simulink model "Idle_Stop_Control"  (R2018a)
settings: configuration reference "Config_Ctrl_Module" (kept outside this file)
PreLoadFcn:
  | HEV_Ctrl_V1_PreLoad
libraries: simulink x1
settings Model: DataDictionary=HEV_Ctrl_V1_Local_data.sldd  Creator=IAEC nishito  LastModifiedBy=E00026

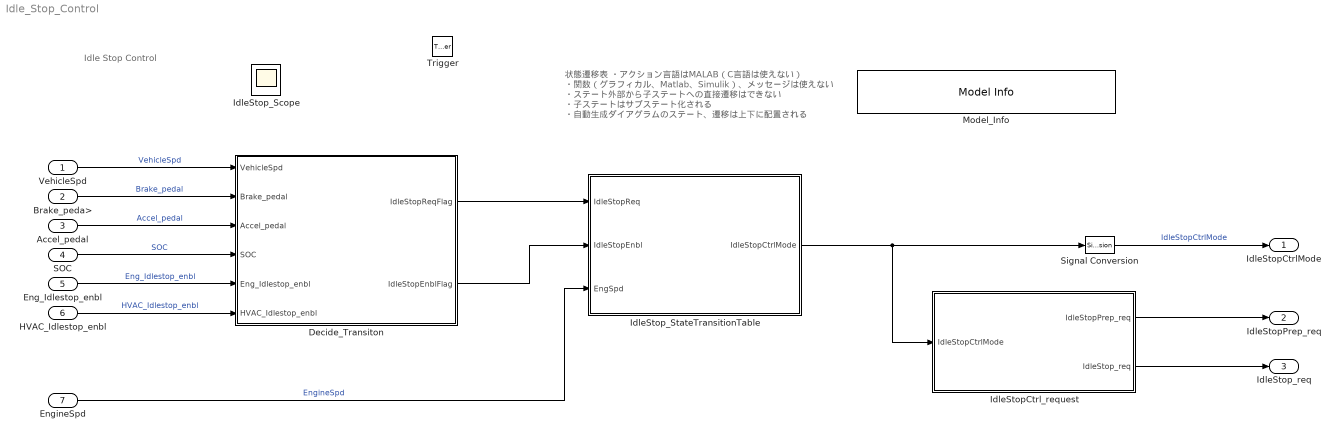
== system Idle_Stop_Control ==
  note: 状態遷移表
      | ・アクション言語はMALAB（C言語は使えない）
      | ・関数（グラフィカル、Matlab、Simulik）、メッセージは使えない
      | ・ステート外部から子ステートへの直接遷移はできない
      | ・子ステートはサブステート化される
      | ・自動生成ダイアグラムのステート、遷移は上下に配置される
  note: Idle Stop Control
  VehicleSpd : Inport  RequirementInfo={} %GIDa_72f7735f_1861_41c0_a3c3_402e3e844fc1  OutDataTypeStr=double  PortDimensions=1
  Brake_peda> : Inport  RequirementInfo={} %GIDa_eb069480_9703_4585_8fff_a42166b4aebb  Port=2  OutDataTypeStr=double  PortDimensions=1
  Accel_pedal : Inport  RequirementInfo={} %GIDa_c2aa2f20_ded1_4ed8_bb49_4c61baf6c527  Port=3  OutDataTypeStr=double  PortDimensions=1
  SOC : Inport  RequirementInfo={} %GIDa_2288a541_41c6_47f0_af5b_526a61592d01  Port=4  OutDataTypeStr=double  PortDimensions=1
  Eng_Idlestop_enbl : Inport  RequirementInfo={} %GIDa_52f2a631_deee_4b81_b109_144a38fb1d39  Port=5  OutDataTypeStr=boolean  PortDimensions=1
  HVAC_Idlestop_enbl : Inport  RequirementInfo={} %GIDa_a5979ef4_7306_49ba_b132_d6093500969e  Port=6  OutDataTypeStr=boolean  PortDimensions=1
  EngineSpd : Inport  RequirementInfo={} %GIDa_0144a9fc_2fd0_4446_b957_811392ba3fbb  Port=7  OutDataTypeStr=double  PortDimensions=1
  Trigger : TriggerPort  RequirementInfo={} %GIDa_12d1da28_9432_4f31_ab1a_c0ce181fbae1  TriggerType=function-call  VariantControl=Variant  PortDimensions=1  TriggerSignalSampleTime=[0.01,0]
  Decide_Transiton : Subsystem  RequirementInfo={} %GIDa_0f8c3e68_9d09_4b6b_9107_8d1ed7fa0379
  IdleStopCtrl_request : Subsystem  RequirementInfo={} %GIDa_43d550b6_444b_4df2_903c_66ed82cd3cc1
  IdleStop_StateTransitionTable : State Transition Table  RequirementInfo={} %GIDa_4a150023_0398_44b8_a842_f2e371cb155a  TreatAsAtomicUnit=on
  Model_Info : simulink/Model-Wide Utilities/Model Info  Frame=on  DisplayStringWithTags=|  HorizontalTextAlignment=Left  LeftAlignmentValue=0.02
      | Version  %<ModelVersion>
      | LastModifided by %<LastModifiedBy>  Date %<LastModificationDate>
      | Description  %<Description>
  Signal Conversion : SignalConversion  OverrideOpt=off
  IdleStopCtrlMode : Outport  RequirementInfo={} %GIDa_55c5f649_78ac_4ac9_b2e5_0d2ecf0ccf0d  OutDataTypeStr=double  PortDimensions=1
  IdleStopPrep_req : Outport  RequirementInfo={} %GIDa_26006239_a740_4660_838b_7c9264c716dc  Port=2  OutDataTypeStr=boolean  PortDimensions=1
  IdleStop_req : Outport  RequirementInfo={} %GIDa_f6c09664_3b1e_412f_baf0_3722afa6614f  Port=3  OutDataTypeStr=boolean  PortDimensions=1
  IdleStop_Scope : Scope
      settings: RequirementInfo={} %GIDa_1aa572e7_9fb2_4501_b2d6_c4ee76e73ea6
  wires:
  IdleStopCtrl_request/2(IdleStop_req) -> IdleStop_req/1
  IdleStop_StateTransitionTable/1(IdleStopCtrlMode) -> IdleStopCtrl_request/1(IdleStopCtrlMode), Signal Conversion/1
  Decide_Transiton/1(IdleStopReqFlag) -> IdleStop_StateTransitionTable/1(IdleStopReq)
  SOC/1 -> Decide_Transiton/4(SOC)  "SOC"
  HVAC_Idlestop_enbl/1 -> Decide_Transiton/6(HVAC_Idlestop_enbl)  "HVAC_Idlestop_enbl"
  IdleStopCtrl_request/1(IdleStopPrep_req) -> IdleStopPrep_req/1
  Decide_Transiton/2(IdleStopEnblFlag) -> IdleStop_StateTransitionTable/2(IdleStopEnbl)
  Eng_Idlestop_enbl/1 -> Decide_Transiton/5(Eng_Idlestop_enbl)  "Eng_Idlestop_enbl"
  Accel_pedal/1 -> Decide_Transiton/3(Accel_pedal)  "Accel_pedal"
  VehicleSpd/1 -> Decide_Transiton/1(VehicleSpd)  "VehicleSpd"
  Brake_peda>/1 -> Decide_Transiton/2(Brake_pedal)  "Brake_pedal"
  EngineSpd/1 -> IdleStop_StateTransitionTable/3(EngSpd)  "EngineSpd"
  Signal Conversion/1 -> IdleStopCtrlMode/1  "IdleStopCtrlMode"

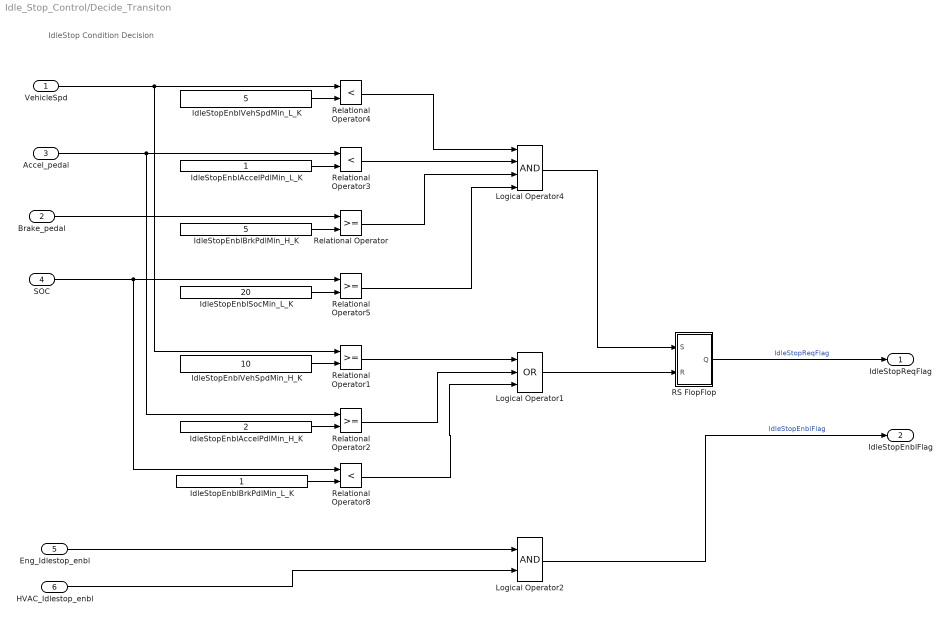
== system Idle_Stop_Control/Decide_Transiton ==
  note: IdleStop Condition Decision
  VehicleSpd : Inport  RequirementInfo={} %GIDa_2ab10adb_7032_4a2c_97a1_7bb0fb165e5e
  Brake_pedal : Inport  RequirementInfo={} %GIDa_47a88e33_5f43_40d8_bc0c_501364992970  Port=2
  Accel_pedal : Inport  RequirementInfo={} %GIDa_fef39789_89f0_45fa_8f85_6b84aa230c69  Port=3
  SOC : Inport  RequirementInfo={} %GIDa_55e6d60a_ee0f_44e0_a38d_ba6e2bf9dbe9  Port=4
  Eng_Idlestop_enbl : Inport  RequirementInfo={} %GIDa_91922d57_691f_49b7_a99e_006b578cf11a  Port=5
  HVAC_Idlestop_enbl : Inport  RequirementInfo={} %GIDa_566c9289_9246_4d35_932c_d372c551c6b7  Port=6
  IdleStopEnblAccelPdlMin_H_K : Constant  RequirementInfo={} %GIDa_806777b1_f885_41a3_adb0_404dc20a194f  Value=2
  IdleStopEnblAccelPdlMin_L_K : Constant  RequirementInfo={} %GIDa_c8f7521b_913c_432c_8051_26ac6e0716a2
  IdleStopEnblBrkPdlMin_H_K : Constant  RequirementInfo={} %GIDa_e5b7d4a4_8bf8_424f_97db_ebec4c30798e  Value=5
  IdleStopEnblBrkPdlMin_L_K : Constant  RequirementInfo={} %GIDa_272b3a83_c857_492d_b6b1_a02b8e962bbe
  IdleStopEnblSocMin_L_K : Constant  RequirementInfo={} %GIDa_3866ca77_8194_43de_88d7_1af354df2f6f  Value=20
  IdleStopEnblVehSpdMin_H_K : Constant  RequirementInfo={} %GIDa_161c09d4_4e2f_45d2_9a9e_7a4b2d014d7d  Value=10
  IdleStopEnblVehSpdMin_L_K : Constant  RequirementInfo={} %GIDa_e4333e70_a7b3_4f07_ad9b_22dc57ba8654  Value=5
  Logical Operator1 : Logic  RequirementInfo={} %GIDa_d1fd0692_7828_4595_92b3_37285b918121  Operator=OR  Inputs=3  AllPortsSameDT=off  OutDataTypeStr=boolean
  Logical Operator2 : Logic  RequirementInfo={} %GIDa_eeb31a4b_771d_490c_936b_5a131afa7c1f  AllPortsSameDT=off  OutDataTypeStr=boolean
  Logical Operator4 : Logic  RequirementInfo={} %GIDa_3a26ed1d_1d0a_42f0_8160_5b4b9b82dbe0  Inputs=4  AllPortsSameDT=off  OutDataTypeStr=boolean
  RS FlopFlop : Subsystem  RequirementInfo={} %GIDa_1f11bf5d_841d_4e55_8521_3cd2fe287deb
  Relational Operator : RelationalOperator  RequirementInfo={} %GIDa_fbc19323_8ea8_455f_abaf_2d6731ecb0a1  OutDataTypeStr=boolean  RndMeth=Nearest
  Relational Operator1 : RelationalOperator  RequirementInfo={} %GIDa_0f689cbf_b206_45df_8702_d5c355afebcd  OutDataTypeStr=boolean  RndMeth=Nearest
  Relational Operator2 : RelationalOperator  RequirementInfo={} %GIDa_badd182d_40d6_46ba_a742_a480e4b72dfc  OutDataTypeStr=boolean  RndMeth=Nearest
  Relational Operator3 : RelationalOperator  RequirementInfo={} %GIDa_9893dff2_f141_4666_ae75_117eb5370ef1  Operator=<  OutDataTypeStr=boolean  RndMeth=Nearest
  Relational Operator4 : RelationalOperator  RequirementInfo={} %GIDa_8927ae18_2ea7_4178_b421_484c846f4f3f  Operator=<  OutDataTypeStr=boolean  RndMeth=Nearest
  Relational Operator5 : RelationalOperator  RequirementInfo={} %GIDa_4427b0fb_90c4_45ec_83a1_a4700bbd409b  OutDataTypeStr=boolean  RndMeth=Nearest
  Relational Operator8 : RelationalOperator  RequirementInfo={} %GIDa_d6849958_8b19_4562_b9e4_7d2057c59388  Operator=<  OutDataTypeStr=boolean  RndMeth=Nearest
  IdleStopReqFlag : Outport  RequirementInfo={} %GIDa_9411fa9e_6f2a_4c7c_909d_f494b4c4f2c2
  IdleStopEnblFlag : Outport  RequirementInfo={} %GIDa_7a1f6d7a_c541_4108_a0bc_a841b5b25c82  Port=2
  wires:
  HVAC_Idlestop_enbl/1 -> Logical Operator2/2
  Eng_Idlestop_enbl/1 -> Logical Operator2/1
  Logical Operator2/1 -> IdleStopEnblFlag/1  "IdleStopEnblFlag"
  IdleStopEnblAccelPdlMin_L_K/1 -> Relational Operator3/2
  Relational Operator5/1 -> Logical Operator4/4
  SOC/1 -> Relational Operator5/1, Relational Operator8/1
  Relational Operator2/1 -> Logical Operator1/2
  IdleStopEnblAccelPdlMin_H_K/1 -> Relational Operator2/2
  Logical Operator4/1 -> RS FlopFlop/1(S)
  IdleStopEnblVehSpdMin_L_K/1 -> Relational Operator4/2
  VehicleSpd/1 -> Relational Operator4/1, Relational Operator1/1
  RS FlopFlop/1(Q) -> IdleStopReqFlag/1  "IdleStopReqFlag"
  IdleStopEnblSocMin_L_K/1 -> Relational Operator5/2
  Accel_pedal/1 -> Relational Operator2/1, Relational Operator3/1
  Relational Operator/1 -> Logical Operator4/3
  IdleStopEnblBrkPdlMin_H_K/1 -> Relational Operator/2
  Brake_pedal/1 -> Relational Operator/1
  Relational Operator4/1 -> Logical Operator4/1
  Relational Operator3/1 -> Logical Operator4/2
  Logical Operator1/1 -> RS FlopFlop/2(R)
  IdleStopEnblVehSpdMin_H_K/1 -> Relational Operator1/2
  IdleStopEnblBrkPdlMin_L_K/1 -> Relational Operator8/2
  Relational Operator1/1 -> Logical Operator1/1
  Relational Operator8/1 -> Logical Operator1/3

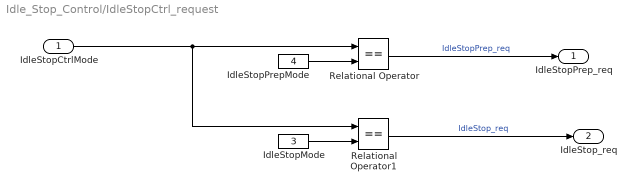
== system Idle_Stop_Control/IdleStopCtrl_request ==
  IdleStopCtrlMode : Inport  RequirementInfo={} %GIDa_1f284967_020f_4205_9752_6dfdc9c13a06
  IdleStopMode : Constant  RequirementInfo={} %GIDa_5e0ca651_d1c8_4f9d_9420_69ebc9aafafb  Value=3
  IdleStopPrepMode : Constant  RequirementInfo={} %GIDa_413a497d_dce0_4397_8719_5d8fd05e37eb  Value=4
  Relational Operator : RelationalOperator  RequirementInfo={} %GIDa_9d9c37b5_ea2b_406f_8f3d_fb66169759d4  Operator===  OutDataTypeStr=boolean  RndMeth=Simplest
  Relational Operator1 : RelationalOperator  RequirementInfo={} %GIDa_1724a5ed_5dcb_4ffd_b16b_83fc4d24ff06  Operator===  OutDataTypeStr=boolean  RndMeth=Simplest
  IdleStopPrep_req : Outport  RequirementInfo={} %GIDa_c88fe8dc_128e_4808_9ef1_67c706cdd285
  IdleStop_req : Outport  RequirementInfo={} %GIDa_88ed3775_e262_4a57_a1cf_ae30085eac21  Port=2
  wires:
  IdleStopPrepMode/1 -> Relational Operator/2
  Relational Operator/1 -> IdleStopPrep_req/1  "IdleStopPrep_req"
  IdleStopMode/1 -> Relational Operator1/2
  IdleStopCtrlMode/1 -> Relational Operator/1, Relational Operator1/1
  Relational Operator1/1 -> IdleStop_req/1  "IdleStop_req"

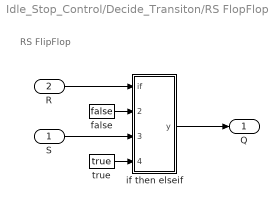
== system Idle_Stop_Control/Decide_Transiton/RS FlopFlop ==
  note: RS FlipFlop
  S : Inport  RequirementInfo={} %GIDa_0a6200b1_c4a0_4772_b261_301d0d627c45
  R : Inport  RequirementInfo={} %GIDa_6e1f103a_7746_4c5c_8128_9c2665cc449d  Port=2
  false : Constant  RequirementInfo={} %GIDa_b8d1b9da_7624_4755_882e_ea884b51896b  Value=false
  if then elseif : Subsystem  RequirementInfo={} %GIDa_b2bf0fbb_ebdd_4d78_ae41_ec1a71f47043  mask(if then elseif){}
  true : Constant  RequirementInfo={} %GIDa_feb0358c_0403_4a1b_8a43_a4add1c7c9f4  Value=true
  Q : Outport  RequirementInfo={} %GIDa_30c2e6ea_c9e6_431a_83b1_8a2226066ab0
  wires:
  S/1 -> if then elseif/3(elseif)
  R/1 -> if then elseif/1(if)
  if then elseif/1(y) -> Q/1
  false/1 -> if then elseif/2(then1)
  true/1 -> if then elseif/4(then2)

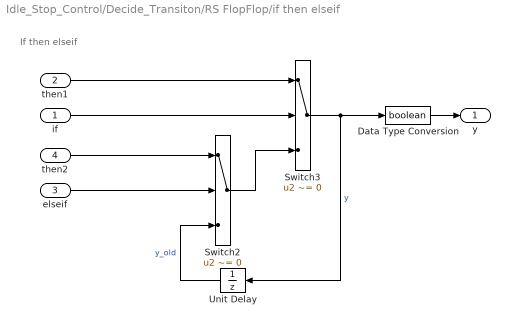
== system Idle_Stop_Control/Decide_Transiton/RS FlopFlop/if then elseif ==
  note: If then elseif
  if : Inport  RequirementInfo={} %GIDa_a06445fc_5d96_4bb4_b90a_65ade8082873
  then1 : Inport  RequirementInfo={} %GIDa_793bcde2_ca84_4662_961f_9b99bee5138c  Port=2
  elseif : Inport  RequirementInfo={} %GIDa_3058ce07_9bdf_4832_8ef2_ce84ef01be25  Port=3
  then2 : Inport  RequirementInfo={} %GIDa_fd0e4a57_410b_4495_b647_ecf5be5ab035  Port=4
  Data Type Conversion : DataTypeConversion  RequirementInfo={} %GIDa_04e57f06_0282_4d92_a01d_4e1bec4290de  OutDataTypeStr=boolean
  Switch2 : Switch  RequirementInfo={} %GIDa_1351dd5c_486a_460b_ba05_1fbf138bbcb6  Criteria=u2 ~= 0  Threshold=0.5  SaturateOnIntegerOverflow=on
      settings: AttributesFormatString=<%<Criteria>>
  Switch3 : Switch  RequirementInfo={} %GIDa_4fa8a9f2_3ad9_4cc8_bb0d_ea07fea45472  Criteria=u2 ~= 0  Threshold=0.5  SaturateOnIntegerOverflow=on
      settings: AttributesFormatString=<%<Criteria>>
  Unit Delay : UnitDelay  RequirementInfo={} %GIDa_94b45ce3_2546_4a04_8f73_a58228ae89e6  SampleTime=-1
      settings: AttributesFormatString=<initial=%<X0>>\n<tsample=%<SampleTime>>
  y : Outport  RequirementInfo={} %GIDa_4d4551a4_f4ea_480d_b486_6b8dd17e1939
  wires:
  Data Type Conversion/1 -> y/1
  Switch2/1 -> Switch3/3
  if/1 -> Switch3/2
  Unit Delay/1 -> Switch2/3  "y_old"
  Switch3/1 -> Data Type Conversion/1, Unit Delay/1  "y"
  then1/1 -> Switch3/1
  elseif/1 -> Switch2/2
  then2/1 -> Switch2/1

== stateflow chart Idle_Stop_Control/IdleStop_StateTransitionTable ==
  state EngineStop
    en:
    IdleStopCtrlMode=0;
  state IdleStop
    en:
    IdleStopCtrlMode=1;
  state EngineStart_Tran
    en:
    IdleStopCtrlMode=2;
  state IdleStopWait_Tran
    en:
    IdleStopCtrlMode=3;
  state IdleStopPrepare
    en:
    IdleStopCtrlMode=4;
  state EngineRun
    en:
    IdleStopCtrlMode=5;
  (default) -> EngineStop
  (junction 32) -> EngineStop
  (junction 52) -> (junction 32)
  EngineStop -> (junction 70) : [EngSpd>300]% Engine run cond
  (junction 70) -> (junction 28)
  (junction 65) -> IdleStop
  (junction 67) -> (junction 65)
  IdleStop -> EngineStart_Tran : [~IdleStopReq]% IdleStop end cond.
  EngineStart_Tran -> IdleStop [order 2] : [IdleStopReq]% IdleStop restart cond.
  EngineStart_Tran -> (junction 28) [order 1] : [EngSpd>300]% Engine run cond
  (junction 28) -> (junction 26)
  IdleStopWait_Tran -> (junction 67) [order 1] : [EngSpd<50]% IdlaStopStartCond.
  IdleStopWait_Tran -> IdleStopPrepare [order 2] : [~IdleStopEnbl || ~IdleStopReq]% IdleStop cancel cond.
  IdleStopPrepare -> IdleStopWait_Tran [order 2] : [IdleStopEnbl && IdleStopCtrlEnbl_K]% IdleStop wait cond.
  IdleStopPrepare -> (junction 52) [order 3] : [EngSpd<50]% Engine stop cond.
  (junction 48) -> (junction 52)
  IdleStopPrepare -> EngineRun [order 1] : [~IdleStopReq]% IdleStop cancel cond.
  EngineRun -> IdleStopPrepare [order 1] : [IdleStopReq]% IdleStop prepare cond.
  EngineRun -> (junction 48) [order 2] : [EngSpd<50]% Engine stop cond.
  (junction 26) -> EngineRun
  data: IdleStopReq input; IdleStopEnbl input; EngSpd input; IdleStopCtrlMode output; IdleStopCtrlEnbl_K parameter
